simulink model "coluna_sim_multiloop"  (R2025a)
settings: Solver=VariableStepAuto  StartTime=0.0  StopTime=3000  RelTol=1e-3
undefined symbols (not defined in the file or in its folder): p
libraries: slpidlib x2
settings Model: Creator=hdafg  LastModifiedBy=hdafg
settings DataIOCC: ExternalInput=inputSignal  OutputSaveName=simData
settings DebuggingCC: BusObjectLabelMismatch=none

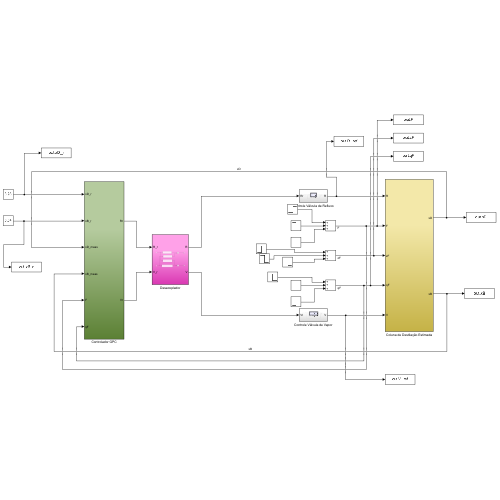
[thumbnail: Simulink's stored preview of the top-level diagram]
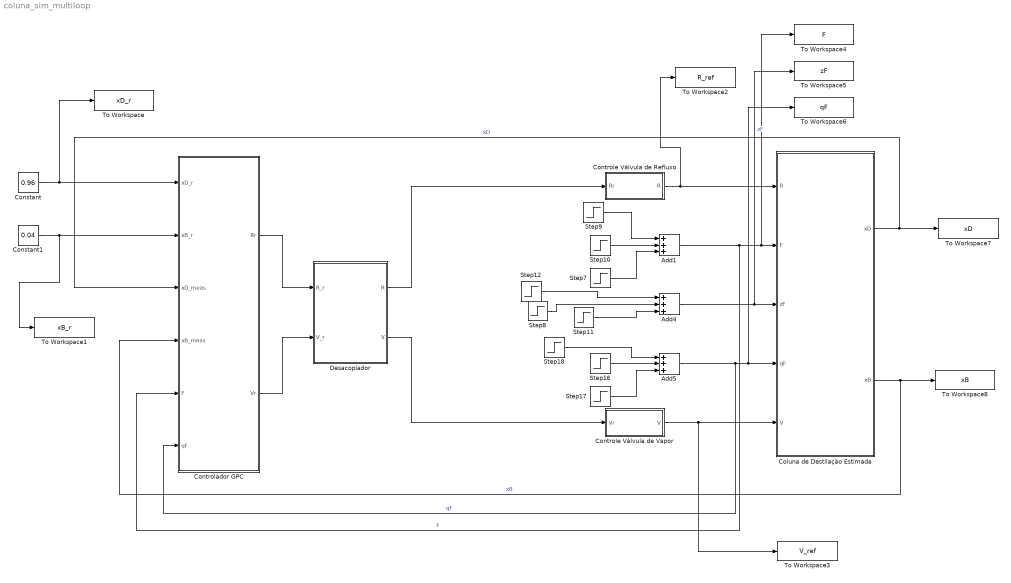
== system coluna_sim_multiloop ==
  Add1 : Sum  Inputs=+++
  Add4 : Sum  Inputs=+++
  Add5 : Sum  Inputs=+++
  Coluna de Destilação Estimada : Subsystem
  Constant : Constant  Value=0.96
  Constant1 : Constant  Value=0.04
  Controlador GPC : Subsystem
  Controle Válvula de Refluxo : Subsystem
  Controle Válvula de Vapor : Subsystem
  Desacoplador : Subsystem
  Step10 : Step  Time=700  After=-0.1  SampleTime=0
  Step11 : Step  Time=1600  After=-0.05  SampleTime=0
  Step12 : Step  Time=1200  Before=0.5  After=0.55  SampleTime=0
  Step16 : Step  Time=2000  After=0.1  SampleTime=0
  Step17 : Step  Time=2200  After=0.1  SampleTime=0
  Step18 : Step  Time=1800  Before=1  After=0.9  SampleTime=0
  Step7 : Step  Time=900  After=-0.1  SampleTime=0
  Step8 : Step  Time=1400  After=-0.05  SampleTime=0
  Step9 : Step  Time=500  Before=1  After=1.1  SampleTime=0
  To Workspace : ToWorkspace  VariableName=xD_r  SaveFormat=Timeseries  SampleTime=-1
  To Workspace1 : ToWorkspace  VariableName=xB_r  SaveFormat=Timeseries  SampleTime=-1
  To Workspace2 : ToWorkspace  VariableName=R_ref  SaveFormat=Timeseries  SampleTime=-1
  To Workspace3 : ToWorkspace  VariableName=V_ref  SaveFormat=Timeseries  SampleTime=-1
  To Workspace4 : ToWorkspace  VariableName=F  SaveFormat=Timeseries  SampleTime=-1
  To Workspace5 : ToWorkspace  VariableName=zF  SaveFormat=Timeseries  SampleTime=-1
  To Workspace6 : ToWorkspace  VariableName=qF  SaveFormat=Timeseries  SampleTime=-1
  To Workspace7 : ToWorkspace  VariableName=xD  SaveFormat=Timeseries  SampleTime=-1
  To Workspace8 : ToWorkspace  VariableName=xB  SaveFormat=Timeseries  SampleTime=-1
  wires:
  Coluna de Destilação Estimada/1(xD) -> To Workspace7/1, Controlador GPC/3(xD_meas)  "xD"
  Coluna de Destilação Estimada/2(xB) -> Controlador GPC/4(xB_meas), To Workspace8/1  "xB"
  Controle Válvula de Vapor/1(V) -> To Workspace3/1, Coluna de Destilação Estimada/5(V)
  Controle Válvula de Refluxo/1(R) -> To Workspace2/1, Coluna de Destilação Estimada/1(R)
  Add1/1 -> Controlador GPC/5(F), To Workspace4/1, Coluna de Destilação Estimada/2(F)  "F"
  Add4/1 -> To Workspace5/1, Coluna de Destilação Estimada/3(zF)  "zF"
  Add5/1 -> Controlador GPC/6(qF), To Workspace6/1, Coluna de Destilação Estimada/4(qF)  "qF"
  Constant/1 -> To Workspace/1, Controlador GPC/1(xD_r)
  Constant1/1 -> To Workspace1/1, Controlador GPC/2(xB_r)
  Controlador GPC/2(Vr) -> Desacoplador/2(V_r)
  Controlador GPC/1(Rr) -> Desacoplador/1(R_r)
  Desacoplador/2(V) -> Controle Válvula de Vapor/1(Vr)
  Desacoplador/1(R) -> Controle Válvula de Refluxo/1(Rr)
  Step17/1 -> Add5/3
  Step12/1 -> Add4/1
  Step8/1 -> Add4/2
  Step10/1 -> Add1/2
  Step9/1 -> Add1/1
  Step16/1 -> Add5/2
  Step7/1 -> Add1/3
  Step18/1 -> Add5/1
  Step11/1 -> Add4/3

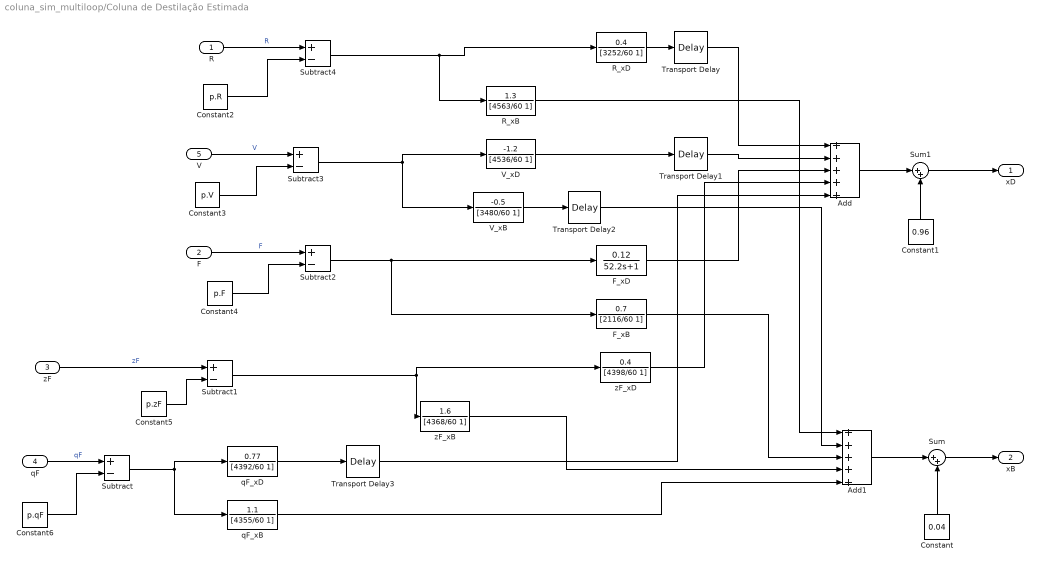
== system coluna_sim_multiloop/Coluna de Destilação Estimada ==
  R : Inport
  F : Inport  Port=2
  zF : Inport  Port=3
  qF : Inport  Port=4
  V : Inport  Port=5
  Add : Sum  Inputs=+++++
  Add1 : Sum  Inputs=+++++
  Constant : Constant  Value=0.04
  Constant1 : Constant  Value=0.96
  Constant2 : Constant  Value=p.R
  Constant3 : Constant  Value=p.V
  Constant4 : Constant  Value=p.F
  Constant5 : Constant  Value=p.zF
  Constant6 : Constant  Value=p.qF
  F_xB : TransferFcn  Numerator=0.7  Denominator=[2116/60 1]
  F_xD : TransferFcn  Numerator=0.12  Denominator=[52.2 1]
  R_xB : TransferFcn  Numerator=1.3  Denominator=[4563/60 1]
  R_xD : TransferFcn  Numerator=[0.4]  Denominator=[3252/60 1]
  Subtract{,1..4} (5 alike) : Sum  Inputs=+-
  Sum : Sum  Inputs=|++
  Sum1 : Sum  Inputs=|++
  Transport Delay : TransportDelay  DelayTime=9.36/60
  Transport Delay1 : TransportDelay  DelayTime=9.6/60
  Transport Delay2 : TransportDelay  DelayTime=9.6
  Transport Delay3 : TransportDelay  DelayTime=17.1/60
  V_xB : TransferFcn  Numerator=-0.5  Denominator=[3480/60 1]
  V_xD : TransferFcn  Numerator=-1.2  Denominator=[4536/60 1]
  qF_xB : TransferFcn  Numerator=1.1  Denominator=[4355/60 1]
  qF_xD : TransferFcn  Numerator=0.77  Denominator=[4392/60 1]
  zF_xB : TransferFcn  Numerator=1.6  Denominator=[4368/60 1]
  zF_xD : TransferFcn  Numerator=0.4  Denominator=[4398/60 1]
  xD : Outport
  xB : Outport  Port=2
  wires:
  F/1 -> Subtract2/1  "F"
  zF/1 -> Subtract1/1  "zF"
  R_xD/1 -> Transport Delay/1
  V_xD/1 -> Transport Delay1/1
  F_xD/1 -> Add/3
  zF_xD/1 -> Add/4
  qF_xD/1 -> Transport Delay3/1
  R_xB/1 -> Add1/1
  V_xB/1 -> Transport Delay2/1
  F_xB/1 -> Add1/3
  zF_xB/1 -> Add1/4
  qF_xB/1 -> Add1/5
  Add1/1 -> Sum/1
  Sum/1 -> xB/1
  Constant/1 -> Sum/2
  Add/1 -> Sum1/1
  Sum1/1 -> xD/1
  Constant1/1 -> Sum1/2
  Transport Delay/1 -> Add/1
  Transport Delay1/1 -> Add/2
  Transport Delay2/1 -> Add1/2
  Transport Delay3/1 -> Add/5
  qF/1 -> Subtract/1  "qF"
  Subtract/1 -> qF_xB/1, qF_xD/1
  Subtract1/1 -> zF_xB/1, zF_xD/1
  Subtract2/1 -> F_xB/1, F_xD/1
  V/1 -> Subtract3/1  "V"
  Subtract3/1 -> V_xB/1, V_xD/1
  R/1 -> Subtract4/1  "R"
  Subtract4/1 -> R_xB/1, R_xD/1
  Constant2/1 -> Subtract4/2
  Constant3/1 -> Subtract3/2
  Constant4/1 -> Subtract2/2
  Constant5/1 -> Subtract1/2
  Constant6/1 -> Subtract/2

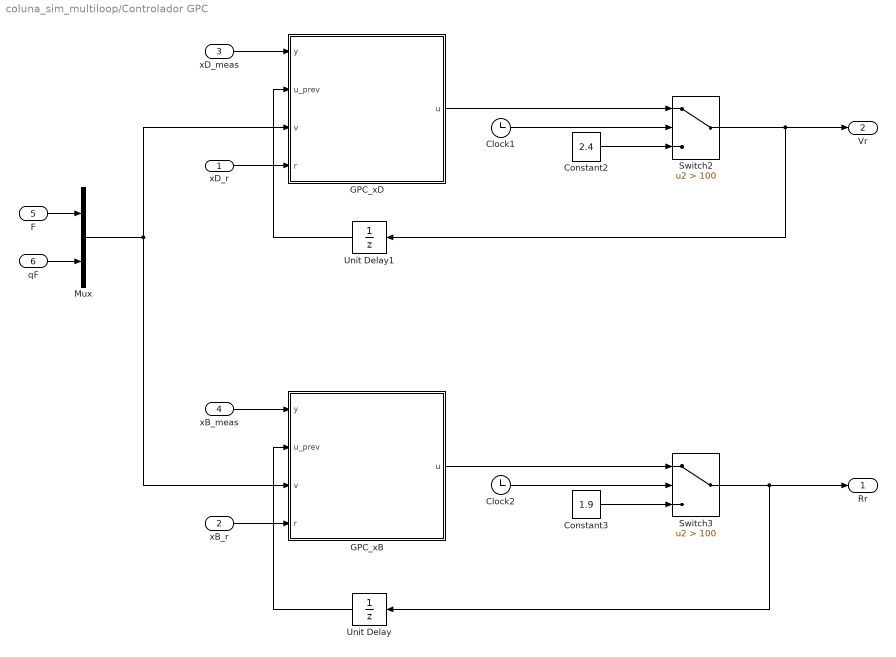
== system coluna_sim_multiloop/Controlador GPC ==
  xD_r : Inport
  xB_r : Inport  Port=2
  xD_meas : Inport  Port=3
  xB_meas : Inport  Port=4
  F : Inport  Port=5
  qF : Inport  Port=6
  Clock1 : Clock
  Clock2 : Clock
  Constant2 : Constant  Value=2.4
  Constant3 : Constant  Value=1.9
  GPC_xB : MATLAB Function  TreatAsAtomicUnit=on
  GPC_xD : MATLAB Function  TreatAsAtomicUnit=on
  Mux : Mux  Inputs=2
  Switch2 : Switch  Criteria=u2 > Threshold  Threshold=100  SaturateOnIntegerOverflow=off  InputSameDT=off
  Switch3 : Switch  Criteria=u2 > Threshold  Threshold=100  SaturateOnIntegerOverflow=off  InputSameDT=off
  Unit Delay : UnitDelay  SampleTime=10  HasFrameUpgradeWarning=on
  Unit Delay1 : UnitDelay  SampleTime=10  HasFrameUpgradeWarning=on
  Rr : Outport
  Vr : Outport  Port=2
  wires:
  xB_r/1 -> GPC_xB/4(r)
  xD_r/1 -> GPC_xD/4(r)
  xD_meas/1 -> GPC_xD/1(y)
  xB_meas/1 -> GPC_xB/1(y)
  Switch2/1 -> Unit Delay1/1, Vr/1
  Constant2/1 -> Switch2/3
  Clock1/1 -> Switch2/2
  Constant3/1 -> Switch3/3
  Switch3/1 -> Unit Delay/1, Rr/1
  GPC_xB/1(u) -> Switch3/1
  GPC_xD/1(u) -> Switch2/1
  Clock2/1 -> Switch3/2
  Unit Delay/1 -> GPC_xB/2(u_prev)
  Unit Delay1/1 -> GPC_xD/2(u_prev)
  qF/1 -> Mux/2
  F/1 -> Mux/1
  Mux/1 -> GPC_xD/3(v), GPC_xB/3(v)

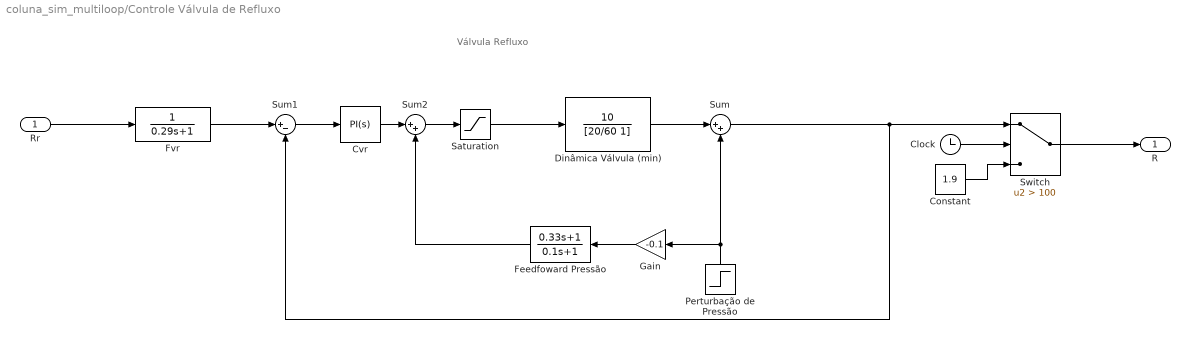
== system coluna_sim_multiloop/Controle Válvula de Refluxo ==
  note: Válvula Refluxo
  Rr : Inport
  Clock : Clock
  Constant : Constant  Value=1.9
  Cvr : slpidlib/PID Controller  Controller=PI  Form=Parallel  TimeDomain=Continuous-time  UseExternalTs=off  SampleTime=-1  IntegratorMethod=Forward Euler  FilterMethod=Forward Euler  ControllerParametersSource=internal  P=0.22  I=0.768  UseKiTs=off  D=0  UseExternalDerivativeSource=off  N=100  UseFilter=on  TunerSelectOption=Transfer Function Based (PID Tuner App)  InitialConditionSource=internal  InitialConditionForIntegrator=0  InitialConditionForFilter=0  DifferentiatorICPrevScaledInput=0  ExternalReset=none  TrackingMode=off  Kt=1  LimitOutput=on  SatLimitsSource=internal  UpperSaturationLimit=1  LowerSaturationLimit=0  LinearizeAsGain=on  AntiWindupMode=back-calculation  Kb=1/0.29  LimitIntegrator=off  UpperIntegratorSaturationLimit=inf  LowerIntegratorSaturationLimit=-inf  POutMin=[]  POutMax=[]  IOutMin=[]  IOutMax=[]  DOutMin=[]  DOutMax=[]  NOutMin=[]  NOutMax=[]  SumOutMin=[]  SumOutMax=[]  SaturationOutMin=[]  SaturationOutMax=[]  PParamMin=[]  PParamMax=[]  IParamMin=[]  IParamMax=[]  DParamMin=[]  DParamMax=[]  NParamMin=[]  NParamMax=[]  KbParamMin=[]  KbParamMax=[]  KtParamMin=[]  KtParamMax=[]  KbOutMin=[]  KbOutMax=[]  KtOutMin=[]  KtOutMax=[]  IntegratorOutMin=[]  IntegratorOutMax=[]  FilterOutMin=[]  FilterOutMax=[]  SumI1OutMin=[]  SumI1OutMax=[]  SumI2OutMin=[]  SumI2OutMax=[]  SumI3OutMin=[]  SumI3OutMax=[]  SumI4OutMin=[]  SumI4OutMax=[]  SumDOutMin=[]  SumDOutMax=[]  DifferentiatorOutMin=[]  DifferentiatorOutMax=[]  FilterDiffOutCoefMin=[]  FilterDiffOutCoefMax=[]  ReciprocalOutMin=[]  ReciprocalOutMax=[]  SumDenOutMin=[]  SumDenOutMax=[]  SumNumOutMin=[]  SumNumOutMax=[]  DivideOutMin=[]  DivideOutMax=[]  UdiffTsProdOutMin=[]  UdiffTsProdOutMax=[]  NTsProdOutMin=[]  NTsProdOutMax=[]  UintegralTsProdOutMin=[]  UintegralTsProdOutMax=[]  UngainTsProdOutMin=[]  UngainTsProdOutMax=[]  ClampingZeroOutDataTypeStr=Inherit: Inherit via back propagation  ClampingZeroOutMin=[]  ClampingZeroOutMax=[]  FilterDenConstantOutDataTypeStr=Inherit: Inherit via back propagation  FilterDenConstantOutMin=[]  FilterDenConstantOutMax=[]  PCopyOutDataTypeStr=Inherit: Inherit via back propagation  PCopyOutMin=[]  PCopyOutMax=[]  NCopyOutDataTypeStr=Inherit: Inherit via back propagation  NCopyOutMin=[]  NCopyOutMax=[]  IntegratorContinuousStateAttributes=''  IntegratorStateMustResolveToSignalObject=off  IntegratorRTWStateStorageClass=Auto  FilterContinuousStateAttributes=''  FilterStateMustResolveToSignalObject=off  FilterRTWStateStorageClass=Auto  ParallelPVariant=InternalParameters  IdealPVariant=Disabled  IVariant=InternalParameters  DVariant=Disabled  IntegratorVariant=Continuous  SatVariant=Enabled  AWVariant=BackCalculation  PCopyVariant=Disabled  TRVariant=Disabled  FdbkBlocksVariant=Forward  IdealPFdbkVariant=Disabled  SatFdbkVariant=Disabled  DerivativeFilterVariant=Disabled  NVariant=Disabled  NCopyVariant=Disabled_SignalSpec  FilterICVariant=Disabled  IntegratorICVariant=InternalICs  ExternalResetVariant=Disabled  TRSumVariant=Passthrough  SumFdbkVariant=Disabled  SumVariant=Sum_PI  TsampFilterVariant=InternalTs  TsampNgainVariant=Passthrough  TsampIntegralVariant=Disabled_SignalSpec  ExternalSaturationOutDataTypeStr=Inherit: Same as second input  DerivativeSourceVariant=Disabled  PreIntVariant=InternalPreInt
  Dinâmica Válvula (min) : TransferFcn  Numerator=[10]  Denominator=[20/60 1]
  Feedfoward Pressão : TransferFcn  Numerator=[0.33 1]  Denominator=[0.1 1]
  Fvr : TransferFcn  Denominator=[0.29 1]
  Gain : Gain  Gain=-0.1
  Perturbação de Pressão : Step  Time=10  After=-1  SampleTime=0
  Saturation : Saturate  UpperLimit=1  LowerLimit=0
  Sum : Sum  Inputs=|++
  Sum1 : Sum  Inputs=|+-
  Sum2 : Sum  Inputs=|++
  Switch : Switch  Criteria=u2 > Threshold  Threshold=100  SaturateOnIntegerOverflow=off  InputSameDT=off
  R : Outport
  wires:
  Cvr/1 -> Sum2/1
  Saturation/1 -> Dinâmica Válvula (min)/1
  Feedfoward Pressão/1 -> Sum2/2
  Perturbação de Pressão/1 -> Gain/1, Sum/2
  Sum1/1 -> Cvr/1
  Gain/1 -> Feedfoward Pressão/1
  Dinâmica Válvula (min)/1 -> Sum/1
  Sum2/1 -> Saturation/1
  Fvr/1 -> Sum1/1
  Sum/1 -> Sum1/2, Switch/1
  Rr/1 -> Fvr/1
  Clock/1 -> Switch/2
  Switch/1 -> R/1
  Constant/1 -> Switch/3

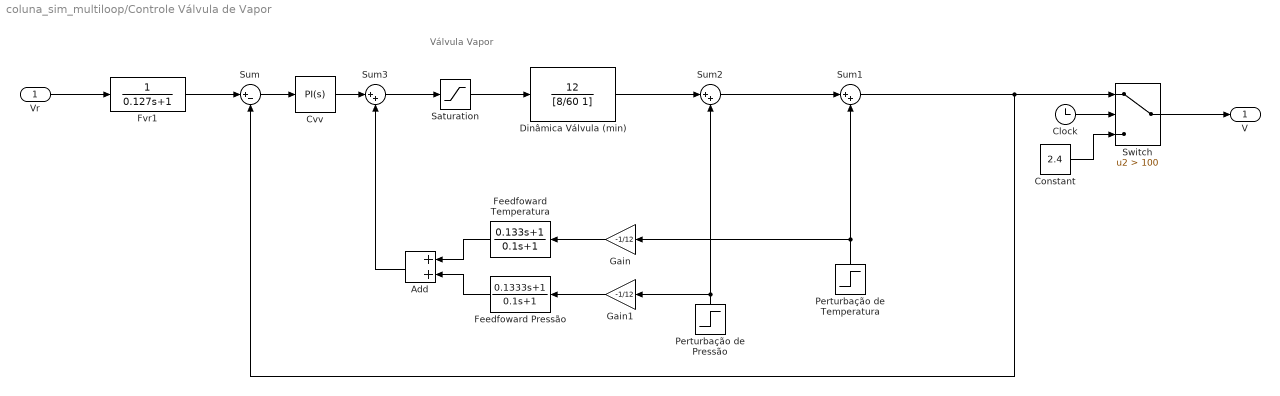
== system coluna_sim_multiloop/Controle Válvula de Vapor ==
  note: Válvula Vapor
  Vr : Inport
  Add : Sum
  Clock : Clock
  Constant : Constant  Value=2.4
  Cvv : slpidlib/PID Controller  Controller=PI  Form=Parallel  TimeDomain=Continuous-time  UseExternalTs=off  SampleTime=-1  IntegratorMethod=Forward Euler  FilterMethod=Forward Euler  ControllerParametersSource=internal  P=0.34  I=2.677  UseKiTs=off  D=0  UseExternalDerivativeSource=off  N=100  UseFilter=on  TunerSelectOption=Transfer Function Based (PID Tuner App)  InitialConditionSource=internal  InitialConditionForIntegrator=0  InitialConditionForFilter=0  DifferentiatorICPrevScaledInput=0  ExternalReset=none  TrackingMode=off  Kt=1  LimitOutput=on  SatLimitsSource=internal  UpperSaturationLimit=1  LowerSaturationLimit=0  LinearizeAsGain=on  AntiWindupMode=back-calculation  Kb=1/0.127  LimitIntegrator=off  UpperIntegratorSaturationLimit=inf  LowerIntegratorSaturationLimit=-inf  POutMin=[]  POutMax=[]  IOutMin=[]  IOutMax=[]  DOutMin=[]  DOutMax=[]  NOutMin=[]  NOutMax=[]  SumOutMin=[]  SumOutMax=[]  SaturationOutMin=[]  SaturationOutMax=[]  PParamMin=[]  PParamMax=[]  IParamMin=[]  IParamMax=[]  DParamMin=[]  DParamMax=[]  NParamMin=[]  NParamMax=[]  KbParamMin=[]  KbParamMax=[]  KtParamMin=[]  KtParamMax=[]  KbOutMin=[]  KbOutMax=[]  KtOutMin=[]  KtOutMax=[]  IntegratorOutMin=[]  IntegratorOutMax=[]  FilterOutMin=[]  FilterOutMax=[]  SumI1OutMin=[]  SumI1OutMax=[]  SumI2OutMin=[]  SumI2OutMax=[]  SumI3OutMin=[]  SumI3OutMax=[]  SumI4OutMin=[]  SumI4OutMax=[]  SumDOutMin=[]  SumDOutMax=[]  DifferentiatorOutMin=[]  DifferentiatorOutMax=[]  FilterDiffOutCoefMin=[]  FilterDiffOutCoefMax=[]  ReciprocalOutMin=[]  ReciprocalOutMax=[]  SumDenOutMin=[]  SumDenOutMax=[]  SumNumOutMin=[]  SumNumOutMax=[]  DivideOutMin=[]  DivideOutMax=[]  UdiffTsProdOutMin=[]  UdiffTsProdOutMax=[]  NTsProdOutMin=[]  NTsProdOutMax=[]  UintegralTsProdOutMin=[]  UintegralTsProdOutMax=[]  UngainTsProdOutMin=[]  UngainTsProdOutMax=[]  ClampingZeroOutDataTypeStr=Inherit: Inherit via back propagation  ClampingZeroOutMin=[]  ClampingZeroOutMax=[]  FilterDenConstantOutDataTypeStr=Inherit: Inherit via back propagation  FilterDenConstantOutMin=[]  FilterDenConstantOutMax=[]  PCopyOutDataTypeStr=Inherit: Inherit via back propagation  PCopyOutMin=[]  PCopyOutMax=[]  NCopyOutDataTypeStr=Inherit: Inherit via back propagation  NCopyOutMin=[]  NCopyOutMax=[]  IntegratorContinuousStateAttributes=''  IntegratorStateMustResolveToSignalObject=off  IntegratorRTWStateStorageClass=Auto  FilterContinuousStateAttributes=''  FilterStateMustResolveToSignalObject=off  FilterRTWStateStorageClass=Auto  ParallelPVariant=InternalParameters  IdealPVariant=Disabled  IVariant=InternalParameters  DVariant=Disabled  IntegratorVariant=Continuous  SatVariant=Enabled  AWVariant=BackCalculation  PCopyVariant=Disabled  TRVariant=Disabled  FdbkBlocksVariant=Forward  IdealPFdbkVariant=Disabled  SatFdbkVariant=Disabled  DerivativeFilterVariant=Disabled  NVariant=Disabled  NCopyVariant=Disabled_SignalSpec  FilterICVariant=Disabled  IntegratorICVariant=InternalICs  ExternalResetVariant=Disabled  TRSumVariant=Passthrough  SumFdbkVariant=Disabled  SumVariant=Sum_PI  TsampFilterVariant=InternalTs  TsampNgainVariant=Passthrough  TsampIntegralVariant=Disabled_SignalSpec  ExternalSaturationOutDataTypeStr=Inherit: Same as second input  DerivativeSourceVariant=Disabled  PreIntVariant=InternalPreInt
  Dinâmica Válvula (min) : TransferFcn  Numerator=[12]  Denominator=[8/60 1]
  Feedfoward Pressão : TransferFcn  Numerator=[0.1333 1]  Denominator=[0.1 1]
  Feedfoward Temperatura : TransferFcn  Numerator=[0.133 1]  Denominator=[0.1 1]
  Fvr1 : TransferFcn  Denominator=[0.127 1]
  Gain : Gain  Gain=-1/12
  Gain1 : Gain  Gain=-1/12
  Perturbação de Pressão : Step  Time=9  After=0.5  SampleTime=0
  Perturbação de Temperatura : Step  Time=12  After=0.8  SampleTime=0
  Saturation : Saturate  UpperLimit=1  LowerLimit=0
  Sum : Sum  Inputs=|+-
  Sum1 : Sum  Inputs=|++
  Sum2 : Sum  Inputs=|++
  Sum3 : Sum  Inputs=|++
  Switch : Switch  Criteria=u2 > Threshold  Threshold=100  SaturateOnIntegerOverflow=off  InputSameDT=off
  V : Outport
  wires:
  Dinâmica Válvula (min)/1 -> Sum2/1
  Feedfoward Pressão/1 -> Add/2
  Perturbação de Pressão/1 -> Sum2/2, Gain1/1
  Sum/1 -> Cvv/1
  Cvv/1 -> Sum3/1
  Add/1 -> Sum3/2
  Feedfoward Temperatura/1 -> Add/1
  Sum1/1 -> Sum/2, Switch/1
  Vr/1 -> Fvr1/1
  Gain1/1 -> Feedfoward Pressão/1
  Saturation/1 -> Dinâmica Válvula (min)/1
  Gain/1 -> Feedfoward Temperatura/1
  Perturbação de Temperatura/1 -> Gain/1, Sum1/2
  Sum3/1 -> Saturation/1
  Sum2/1 -> Sum1/1
  Fvr1/1 -> Sum/1
  Switch/1 -> V/1
  Clock/1 -> Switch/2
  Constant/1 -> Switch/3

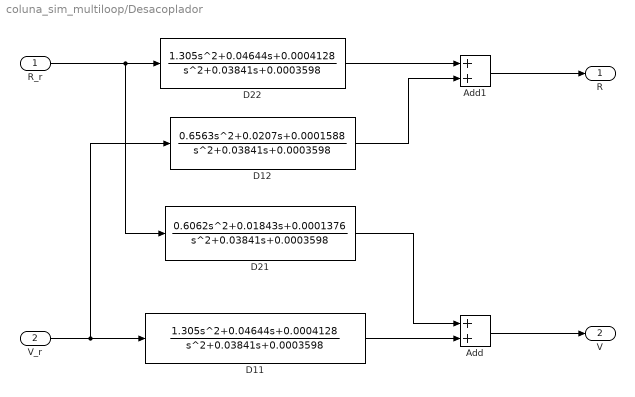
== system coluna_sim_multiloop/Desacoplador ==
  R_r : Inport
  V_r : Inport  Port=2
  Add : Sum
  Add1 : Sum
  D11 : TransferFcn  Numerator=[1.305 0.04644 0.0004128]  Denominator=[1 0.03841 0.0003598]
  D12 : TransferFcn  Numerator=[0.6563 0.0207 0.0001588]  Denominator=[1 0.03841 0.0003598]
  D21 : TransferFcn  Numerator=[0.6062 0.01843 0.0001376]  Denominator=[1 0.03841 0.0003598]
  D22 : TransferFcn  Numerator=[1.305 0.04644 0.0004128]  Denominator=[1 0.03841 0.0003598]
  R : Outport
  V : Outport  Port=2  VectorParamsAs1DForOutWhenUnconnected=off
  wires:
  V_r/1 -> D12/1, D11/1
  Add/1 -> V/1
  R_r/1 -> D21/1, D22/1
  Add1/1 -> R/1
  D11/1 -> Add/2
  D21/1 -> Add/1
  D12/1 -> Add1/2
  D22/1 -> Add1/1

== matlab function coluna_sim_multiloop/Controlador GPC/GPC_xB ==
  settings: updateMethod=DISCRETE  sampleTime=10
  data: y input; u output; u_prev input; v input; r input
function u = GPC_Controller_Block_Loop2(y, u_prev, v, r)
% Bloco de função do GPC (Loop 2: R -> xB)
% Entradas: y(2), u(2)_prev, v (vetor 2x1), r(2)
% Saída: u(2)

%#codegen

% Usar persistent para carregar dados apenas uma vez
persistent controller_data
if isempty(controller_data)
    data = coder.load('GPC_Loop2_Data.mat');
    controller_data = data.controller_data;
end

% Chamar função do controlador
[u, ~, ~] = GPC_SISO_Controller(y, u_prev, v, r, controller_data);

end

== matlab function coluna_sim_multiloop/Controlador GPC/GPC_xD ==
  settings: updateMethod=DISCRETE  sampleTime=10
  data: y input; u output; u_prev input; v input; r input
function u = GPC_Controller_Block_Loop1(y, u_prev, v, r)
% Bloco de função do GPC (Loop 1: V -> xD)
% Entradas: y(1), u(1)_prev, v (vetor 2x1), r(1)
% Saída: u(1)

%#codegen

% Usar persistent para carregar dados apenas uma vez
persistent controller_data
if isempty(controller_data)
    data = coder.load('GPC_Loop1_Data.mat');
    controller_data = data.controller_data;
end

% Chamar função do controlador
[u, ~, ~] = GPC_SISO_Controller(y, u_prev, v, r, controller_data);

end
